simulink model "closed_loop"  (R2020b)
settings: Solver=VariableStepAuto  StartTime=0.0  StopTime=1000  RelTol=1e-3
values from neighbouring files (symbols this model uses):
  A = zeros(size(B'))    [parameters.m]
  Ad = sysd.A    [mpc.m]    (also in parameters.m)
  B = [repmat(eye(3),[1 4]) ... (first row only)    [parameters.m]
  Bd = sysd.B    [mpc.m]    (also in parameters.m)
  I = 4000*eye(3)    [parameters.m]
  K_steer = lqr(Ae,Be,Q,10)    [parameters.m]
  mass = 2000    [parameters.m]
  N = size(R,1)/nStates-1    [body_force_mpc.m]    (also in mpc.m; parameters.m = 10)
  Qf = 1e3*eye(6)    [parameters.m]
  Qu = cost_matrix(Qu,N)    [body_force_mpc.m]    (also in mpc.m; parameters.m = 1e-3*eye(3))
  Qx = blkdiag(cost_matrix(Qx,N-1),Qf)    [body_force_mpc.m]    (also in mpc.m = cost_matrix(Qx,N); parameters.m = eye(6))
  R = R(:)    [body_force_mpc.m]    (also in generate_reference.m = zeros(length(r_0),length(t)); mpc.m; parameters.m = cell2mat(arrayfun(r,tau,'UniformOutput',false)); reference_generator.m = R(:,1:super_sample_ratio:end))
  r_1 = [front_length;width/2;-height]    [parameters.m]
  radius = 0.4    [parameters.m]
  rear_length = 1.6    [parameters.m]
  T = 0.1    [mpc.m]    (also in parameters.m)
  turn_limit = deg2rad(30)    [parameters.m]
  v_0 = 10    [parameters.m]
  width = 2    [parameters.m]
libraries: autolibshared x5, vrlib x4
(part 1 of 4)
settings Model: Creator=Zephyrus  LastModifiedBy=ssa
settings DebuggingCC: SFMachineParentedDataDiag=error

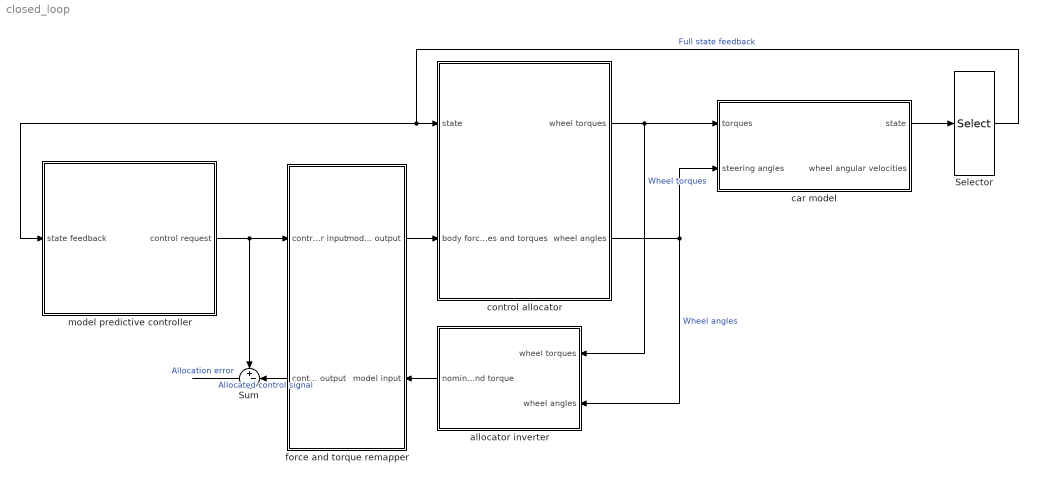
== system closed_loop ==
  Selector : Selector  InputPortWidth=8  IndexOptions=Index vector (dialog)  Indices=[1 2 7 4 5 8]  OutputSizes=1
  Sum : Sum  Inputs=+-|
  allocator inverter : Subsystem
  car model : Subsystem
  control allocator : Subsystem
  force and torque remapper : Subsystem
      settings: PortSchema="{\"entries\":[{\"content\":{\"sides\":[{\"content\":{\"connectorIds\":[\"In1\",\"Out2\"]},\"type\":\"ConnectorPlacement.EquallySpacedRectSide\",\"uuid\":\"d12e0a54-562f-4212-b665-aecd4aa860f9\"},{\"content\":{\"connectorIds\":[\"Out1\",\"In2\"],\"side\":\"RIGHT\"},\"type\":\"ConnectorPlacement.EquallySpacedRectSide\",\"uuid\":\"51912325-17ef-4f81-a98b-a203f2dd415c\"},{\"content\":{\"connectorIds\":[],\"side\":\"TOP\"},\"type\":\"ConnectorPlacement.EquallySpacedRectSide\",\"uuid\":\"d25a9dfd-443b-493f-b5d0-b86de9282602\"},{\"content\":{\"connectorIds\":[],\"side\":\"HIDDEN\"},\"type\":\"ConnectorPlacement.EquallySpacedRectSide\",\"uuid\":\"f66f9800-cfc0-4261-bd5e-1620dcc6560a\"}]},\"type\":\"ConnectorPlacement.EquallySpacedConnector\",\"uuid\":\"ff8a2ae2-42bb-4b93-8940-dc3ccce5b8f6\"}],\"packageUris\":[\"http://schema.mathworks.com/mf0/Connector/R2020b\"],\"version\":\"1.0\"}"
  model predictive controller : Subsystem
  wires:
  control allocator/1(wheel torques) -> car model/1(torques), allocator inverter/1(wheel torques)  "Wheel torques"
  control allocator/2(wheel angles) -> allocator inverter/2(wheel angles), car model/2(steering angles)  "Wheel angles"
  Selector/1 -> control allocator/1(state), model predictive controller/1(state feedback)  "Full state feedback"
  force and torque remapper/1(model output) -> control allocator/2(body forces and torques)
  allocator inverter/1(nominal body force and torque) -> force and torque remapper/2(model input)
  model predictive controller/1(control request) -> Sum/1, force and torque remapper/1(controller input)
  car model/1(state) -> Selector/1
  force and torque remapper/2(controller output) -> Sum/2  "Allocated control signal"
  Sum/1 -> ?  "Allocation error"

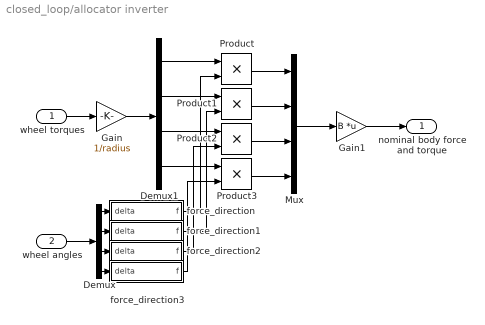
== system closed_loop/allocator inverter ==
  wheel torques : Inport
  wheel angles : Inport  Port=2
  Demux : Demux
  Demux1 : Demux
  Gain : Gain  Gain=1/radius
  Gain1 : Gain  Gain=B  Multiplication=Matrix(K*u)
  Mux : Mux
  Product{,1..3} (4 alike) : Product
  force_direction : MATLAB Function  TreatAsAtomicUnit=on
  force_direction1 : MATLAB Function  TreatAsAtomicUnit=on
  force_direction2 : MATLAB Function  TreatAsAtomicUnit=on
  force_direction3 : MATLAB Function  TreatAsAtomicUnit=on
  nominal body force and torque : Outport
  wires:
  wheel angles/1 -> Demux/1
  Demux/1 -> force_direction/1(delta)
  Demux/2 -> force_direction1/1(delta)
  Demux/3 -> force_direction2/1(delta)
  Demux/4 -> force_direction3/1(delta)
  wheel torques/1 -> Gain/1
  Gain/1 -> Demux1/1
  Demux1/1 -> Product/1
  Demux1/2 -> Product1/1
  Demux1/3 -> Product2/1
  Demux1/4 -> Product3/1
  force_direction3/1(f) -> Product3/2
  force_direction2/1(f) -> Product2/2
  force_direction1/1(f) -> Product1/2
  force_direction/1(f) -> Product/2
  Product/1 -> Mux/1
  Product1/1 -> Mux/2
  Product2/1 -> Mux/3
  Product3/1 -> Mux/4
  Gain1/1 -> nominal body force and torque/1
  Mux/1 -> Gain1/1

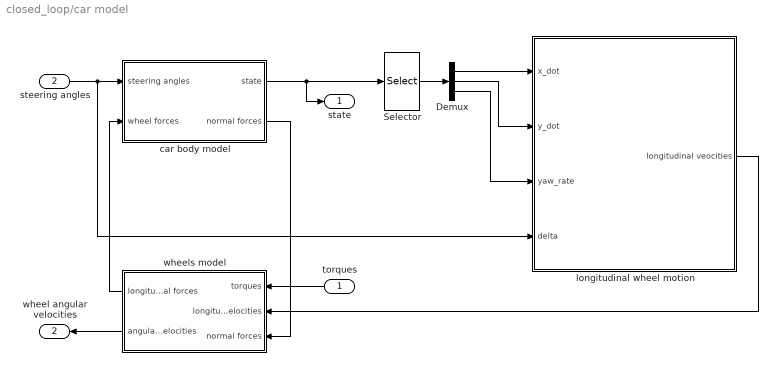
== system closed_loop/car model ==
  torques : Inport
  steering angles : Inport  Port=2
  Demux : Demux  Outputs=3
  Selector : Selector  InputPortWidth=8  IndexOptions=Index vector (dialog)  Indices=[4 5 8]  OutputSizes=1
  car body model : Subsystem
  longitudinal wheel motion : Subsystem
  wheels model : Subsystem
  state : Outport
  wheel angular velocities : Outport  Port=2
  wires:
  car body model/1(state) -> state/1, Selector/1
  Selector/1 -> Demux/1
  Demux/1 -> longitudinal wheel motion/1(x_dot)
  Demux/2 -> longitudinal wheel motion/2(y_dot)
  Demux/3 -> longitudinal wheel motion/3(yaw_rate)
  torques/1 -> wheels model/1(torques)
  steering angles/1 -> car body model/1(steering angles), longitudinal wheel motion/4(delta)
  longitudinal wheel motion/1(longitudinal veocities) -> wheels model/2(longitudinal velocities)
  car body model/2(normal forces) -> wheels model/3(normal forces)
  wheels model/2(angular velocities) -> wheel angular velocities/1
  wheels model/1(longitudinal forces) -> car body model/2(wheel forces)

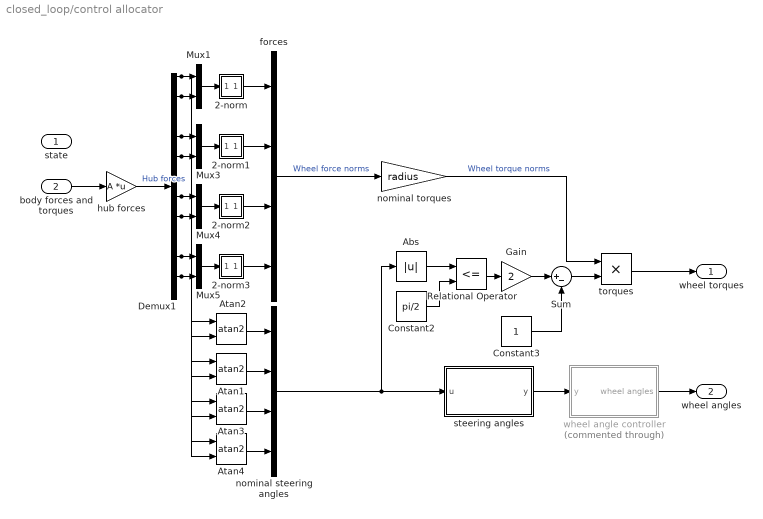
== system closed_loop/control allocator ==
  state : Inport
  body forces and torques : Inport  Port=2
  2-norm : Subsystem
  2-norm1 : Subsystem
  2-norm2 : Subsystem
  2-norm3 : Subsystem
  Abs : Abs
  Atan{1..4} (4 alike) : Trigonometry  Operator=atan2
  Constant2 : Constant  Value=pi/2
  Constant3 : Constant
  Demux1 : Demux  Outputs=12
  Gain : Gain  Gain=2
  Mux{1,3..5} (4 alike) : Mux  Inputs=2
  Relational Operator : RelationalOperator  Operator=<=  OutDataTypeStr=boolean  RndMeth=Simplest
  Sum : Sum  Inputs=|+-
  forces : Mux
  hub forces : Gain  Gain=A  Multiplication=Matrix(K*u)
  nominal steering angles : Mux
  nominal torques : Gain  Gain=radius
  steering angles : MATLAB Function  TreatAsAtomicUnit=on
  torques : Product
  wheel angle controller : Subsystem  Commented=through
  wheel torques : Outport
  wheel angles : Outport  Port=2
  wires:
  hub forces/1 -> Demux1/1  "Hub forces"
  Mux4/1 -> 2-norm2/1(In1)
  Demux1/5 -> Atan1/1, Mux3/2
  Relational Operator/1 -> Gain/1
  Demux1/7 -> Atan3/2, Mux4/1
  Demux1/1 -> Atan2/2, Mux1/1
  Demux1/2 -> Atan2/1, Mux1/2
  Mux3/1 -> 2-norm1/1(In1)
  Atan1/1 -> nominal steering angles/2
  Mux5/1 -> 2-norm3/1(In1)
  Demux1/10 -> Atan4/2, Mux5/1
  Demux1/11 -> Atan4/1, Mux5/2
  Sum/1 -> torques/2
  Demux1/4 -> Atan1/2, Mux3/1
  nominal torques/1 -> torques/1  "Wheel torque norms"
  Demux1/8 -> Atan3/1, Mux4/2
  2-norm2/1(Out1) -> forces/3
  Mux1/1 -> 2-norm/1(In1)
  2-norm1/1(Out1) -> forces/2
  Abs/1 -> Relational Operator/1
  Atan3/1 -> nominal steering angles/3
  2-norm3/1(Out1) -> forces/4
  2-norm/1(Out1) -> forces/1
  Gain/1 -> Sum/1
  Constant2/1 -> Relational Operator/2
  Atan2/1 -> nominal steering angles/1
  forces/1 -> nominal torques/1  "Wheel force norms"
  Constant3/1 -> Sum/2
  torques/1 -> wheel torques/1
  Atan4/1 -> nominal steering angles/4
  nominal steering angles/1 -> Abs/1, steering angles/1(u)
  body forces and torques/1 -> hub forces/1
  steering angles/1(y) -> wheel angle controller/1(y)
  wheel angle controller/1(wheel angles) -> wheel angles/1

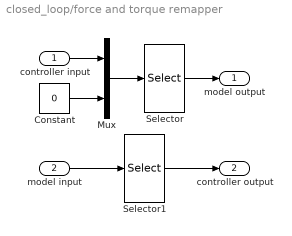
== system closed_loop/force and torque remapper ==
  controller input : Inport
  model input : Inport  Port=2
  Constant : Constant  Value=0
  Mux : Mux  Inputs=2
  Selector : Selector  InputPortWidth=4  IndexOptions=Index vector (dialog)  Indices=[1 2 4 4 4 3]  OutputSizes=1
  Selector1 : Selector  InputPortWidth=6  IndexOptions=Index vector (dialog)  Indices=[1 2 6]  OutputSizes=1
  model output : Outport
  controller output : Outport  Port=2
  wires:
  Mux/1 -> Selector/1
  controller input/1 -> Mux/1
  Constant/1 -> Mux/2
  Selector/1 -> model output/1
  Selector1/1 -> controller output/1
  model input/1 -> Selector1/1

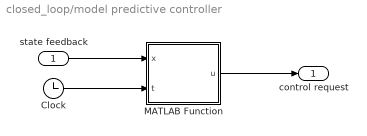
== system closed_loop/model predictive controller ==
  state feedback : Inport
  Clock : Clock
  MATLAB Function : MATLAB Function  TreatAsAtomicUnit=on
  control request : Outport
  wires:
  state feedback/1 -> MATLAB Function/1(x)
  MATLAB Function/1(u) -> control request/1
  Clock/1 -> MATLAB Function/2(t)

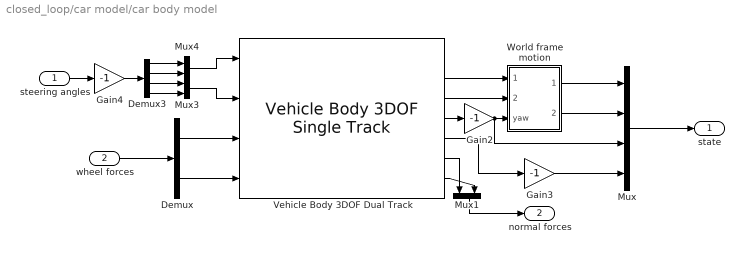
== system closed_loop/car model/car body model ==
  steering angles : Inport
  wheel forces : Inport  Port=2
  Demux : Demux  Outputs=2
  Demux3 : Demux
  Gain2 : Gain  Gain=-1
  Gain3 : Gain  Gain=-1
  Gain4 : Gain  Gain=-1
  Mux : Mux
  Mux1 : Mux  Inputs=2
  Mux3 : Mux  Inputs=2
  Mux4 : Mux  Inputs=2
  Vehicle Body 3DOF Dual Track : autolibshared/Vehicle Body 3DOF Single Track  trackMode=Dual  inputMode=External longitudinal forces  frontSteerMode=on  rearSteerMode=on  windMode=off  muMode=off  extFMode=off  extMMode=off  htchFMode=off  htchMMode=off  extXo=off  extpsio=off  extxdoto=off  extro=off  extYo=off  extTamb=off  extydoto=off  aMode=2  NF=2  NR=2  m=mass  a=front_length  b=rear_length  h=height  dh=1  hh=0.2  X_o=0  xdot_o=v_0  CalphaMode=off  sigmaMode=on  d=0  hl=0  w=[width/2,width/2]  Cy_f=12e3  Cy_r=11e3  sigma_f=.1  sigma_r=.1  alpha_f_brk=[-.1 .1]  Cy_f_data=[-9e3 9e3]  alpha_r_brk=[-.1 .1]  Cy_r_data=[-9e3 9e3]  Y_o=0  ydot_o=0  Izz=I(3,3)  psi_o=0  r_o=0  Af=2  Cd=.3  Cl=.1  Cpm=.1  beta_w=[0:0.01:0.3]  Cs=[0:0.03:0.9]  Cym=[0:0.01:0.3]  Pabs=101325  Tair=273  g=9.81  mu=mu  xdot_tol=.01  Fznom=5000  Fxtire_sat=7e4  Fytire_sat=7e4  longOff=0  latOff=0  vertOff=0  wrapAng=off
      settings: SourceProductBaseCode=PW,DR,MT,UV,VE
  World frame motion : Subsystem
  state : Outport
  normal forces : Outport  Port=2
  wires:
  Vehicle Body 3DOF Dual Track/2 -> World frame motion/1(x_dot)
  World frame motion/1(position) -> Mux/1
  World frame motion/2(velocity) -> Mux/2
  Demux3/1 -> Mux4/1
  Demux3/2 -> Mux4/2
  Demux3/3 -> Mux3/1
  Demux3/4 -> Mux3/2
  Mux4/1 -> Vehicle Body 3DOF Dual Track/1
  Mux3/1 -> Vehicle Body 3DOF Dual Track/2
  Demux/1 -> Vehicle Body 3DOF Dual Track/3
  Demux/2 -> Vehicle Body 3DOF Dual Track/4
  wheel forces/1 -> Demux/1
  Mux/1 -> state/1
  Vehicle Body 3DOF Dual Track/4 -> Gain2/1
  Gain2/1 -> Mux/3, World frame motion/3(yaw)
  Vehicle Body 3DOF Dual Track/3 -> World frame motion/2(y_dot)
  Vehicle Body 3DOF Dual Track/5 -> Gain3/1
  Gain3/1 -> Mux/4
  Vehicle Body 3DOF Dual Track/6 -> Mux1/1
  Vehicle Body 3DOF Dual Track/7 -> Mux1/2
  Mux1/1 -> normal forces/1
  steering angles/1 -> Gain4/1
  Gain4/1 -> Demux3/1

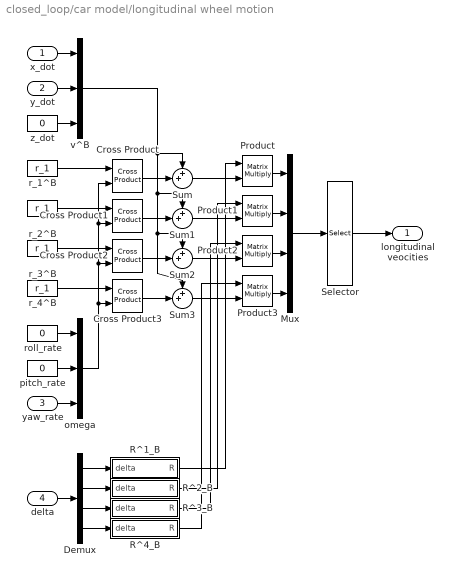
== system closed_loop/car model/longitudinal wheel motion ==
  x_dot : Inport
  y_dot : Inport  Port=2
  yaw_rate : Inport  Port=3
  delta : Inport  Port=4
  Cross Product{,1..3} (4 alike) : vrlib/Utilities/Cross Product
  Demux : Demux
  Mux : Mux
  Product{,1..3} (4 alike) : Product  Multiplication=Matrix(*)
  R^1_B : MATLAB Function  TreatAsAtomicUnit=on
  R^2_B : MATLAB Function  TreatAsAtomicUnit=on
  R^3_B : MATLAB Function  TreatAsAtomicUnit=on
  R^4_B : MATLAB Function  TreatAsAtomicUnit=on
  Selector : Selector  InputPortWidth=12  IndexOptions=Index vector (dialog)  Indices=1:3:12  OutputSizes=1
  Sum{,1..3} (4 alike) : Sum  Inputs=++|
  omega : Mux  Inputs=3
  pitch_rate : Constant  Value=0
  r_1^B : Constant  Value=r_1
  r_2^B : Constant  Value=r_1
  r_3^B : Constant  Value=r_1
  r_4^B : Constant  Value=r_1
  roll_rate : Constant  Value=0
  v^B : Mux  Inputs=3
  z_dot : Constant  Value=0
  longitudinal veocities : Outport
  wires:
  x_dot/1 -> v^B/1
  y_dot/1 -> v^B/2
  z_dot/1 -> v^B/3
  yaw_rate/1 -> omega/3
  roll_rate/1 -> omega/1
  pitch_rate/1 -> omega/2
  r_1^B/1 -> Cross Product/1
  omega/1 -> Cross Product3/2, Cross Product2/2, Cross Product/2, Cross Product1/2
  r_2^B/1 -> Cross Product1/1
  r_3^B/1 -> Cross Product2/1
  r_4^B/1 -> Cross Product3/1
  Cross Product/1 -> Sum/2
  Cross Product1/1 -> Sum1/2
  Cross Product2/1 -> Sum2/2
  Cross Product3/1 -> Sum3/2
  v^B/1 -> Sum/1, Sum1/1, Sum2/1, Sum3/1
  delta/1 -> Demux/1
  Demux/1 -> R^1_B/1(delta)
  Demux/2 -> R^2_B/1(delta)
  Demux/3 -> R^3_B/1(delta)
  Demux/4 -> R^4_B/1(delta)
  Sum/1 -> Product/2
  Sum1/1 -> Product1/2
  Sum2/1 -> Product2/2
  Sum3/1 -> Product3/2
  R^1_B/1(R) -> Product/1
  R^2_B/1(R) -> Product1/1
  R^3_B/1(R) -> Product2/1
  R^4_B/1(R) -> Product3/1
  Product/1 -> Mux/1
  Product3/1 -> Mux/4
  Product1/1 -> Mux/2
  Product2/1 -> Mux/3
  Mux/1 -> Selector/1
  Selector/1 -> longitudinal veocities/1
